simulink model "SVPWM"  (R2022a)
settings: Solver=ode23  StartTime=0.0  StopTime=0.1  MaxStep=1e-5  RelTol=1e-3
libraries: simulink x1
settings Model: Creator=123  LastModifiedBy=123

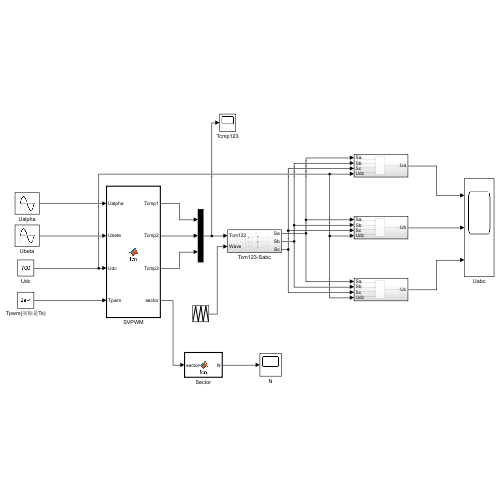
[thumbnail: Simulink's stored preview of the top-level diagram]
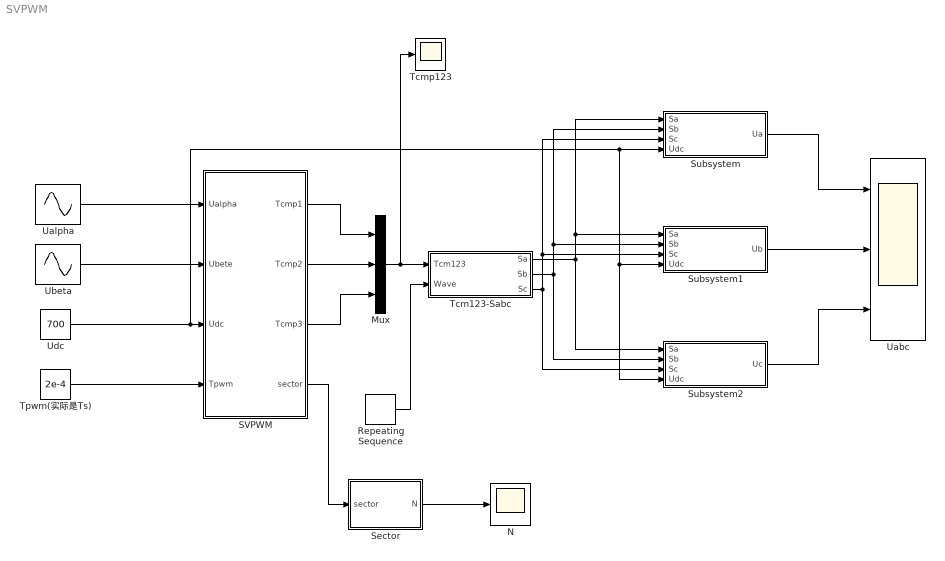
== system SVPWM ==
  Mux : Mux  Inputs=3
  N : Scope
  Repeating Sequence : simulink/Sources/Repeating Sequence  rep_seq_t=[0 0.0001 0.0002]  rep_seq_y=[0 0.0001 0]
  SVPWM : MATLAB Function  TreatAsAtomicUnit=on
  Sector : MATLAB Function  TreatAsAtomicUnit=on
  Subsystem : Subsystem
  Subsystem1 : Subsystem
  Subsystem2 : Subsystem
  Tcm123-Sabc : Subsystem
  Tcmp123 : Scope
  Tpwm(实际是Ts) : Constant  Value=2e-4
  Uabc : Scope  NumInputPorts=3
  Ualpha : Sin  Amplitude=200  Frequency=2*50*pi  Phase=pi/2  SampleTime=0
  Ubeta : Sin  Amplitude=200  Frequency=2*50*pi  SampleTime=0
  Udc : Constant  Value=700
  wires:
  Subsystem/1(Ua) -> Uabc/1
  Subsystem1/1(Ub) -> Uabc/2
  Subsystem2/1(Uc) -> Uabc/3
  Ualpha/1 -> SVPWM/1(Ualpha)
  Ubeta/1 -> SVPWM/2(Ubete)
  Udc/1 -> Subsystem/4(Udc), Subsystem1/4(Udc), Subsystem2/4(Udc), SVPWM/3(Udc)
  Tpwm(实际是Ts)/1 -> SVPWM/4(Tpwm)
  SVPWM/1(Tcmp1) -> Mux/1
  SVPWM/2(Tcmp2) -> Mux/2
  SVPWM/3(Tcmp3) -> Mux/3
  Mux/1 -> Tcmp123/1, Tcm123-Sabc/1(Tcm123)
  Repeating Sequence/1 -> Tcm123-Sabc/2(Wave)
  Tcm123-Sabc/1(Sa) -> Subsystem2/1(Sa), Subsystem1/1(Sa), Subsystem/1(Sa)
  Tcm123-Sabc/2(Sb) -> Subsystem2/2(Sb), Subsystem1/2(Sb), Subsystem/2(Sb)
  Tcm123-Sabc/3(Sc) -> Subsystem2/3(Sc), Subsystem1/3(Sc), Subsystem/3(Sc)
  SVPWM/4(sector) -> Sector/1(sector)
  Sector/1(N) -> N/1

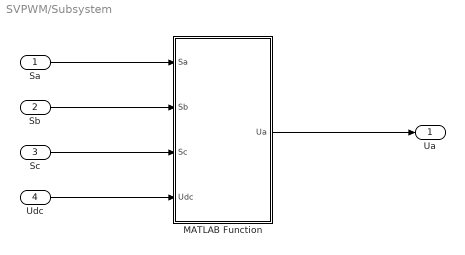
== system SVPWM/Subsystem ==
  Sa : Inport
  Sb : Inport  Port=2
  Sc : Inport  Port=3
  Udc : Inport  Port=4
  MATLAB Function : MATLAB Function  TreatAsAtomicUnit=on
  Ua : Outport
  wires:
  MATLAB Function/1(Ua) -> Ua/1
  Sa/1 -> MATLAB Function/1(Sa)
  Sb/1 -> MATLAB Function/2(Sb)
  Sc/1 -> MATLAB Function/3(Sc)
  Udc/1 -> MATLAB Function/4(Udc)

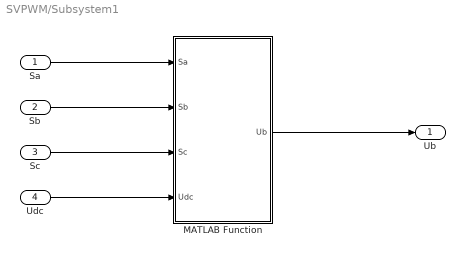
== system SVPWM/Subsystem1 ==
  Sa : Inport
  Sb : Inport  Port=2
  Sc : Inport  Port=3
  Udc : Inport  Port=4
  MATLAB Function : MATLAB Function  TreatAsAtomicUnit=on
  Ub : Outport
  wires:
  Sc/1 -> MATLAB Function/3(Sc)
  Udc/1 -> MATLAB Function/4(Udc)
  Sa/1 -> MATLAB Function/1(Sa)
  Sb/1 -> MATLAB Function/2(Sb)
  MATLAB Function/1(Ub) -> Ub/1

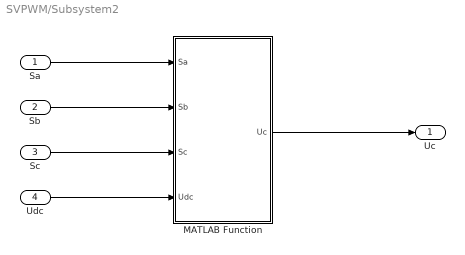
== system SVPWM/Subsystem2 ==
  Sa : Inport
  Sb : Inport  Port=2
  Sc : Inport  Port=3
  Udc : Inport  Port=4
  MATLAB Function : MATLAB Function  TreatAsAtomicUnit=on
  Uc : Outport
  wires:
  Sc/1 -> MATLAB Function/3(Sc)
  Udc/1 -> MATLAB Function/4(Udc)
  Sa/1 -> MATLAB Function/1(Sa)
  Sb/1 -> MATLAB Function/2(Sb)
  MATLAB Function/1(Uc) -> Uc/1

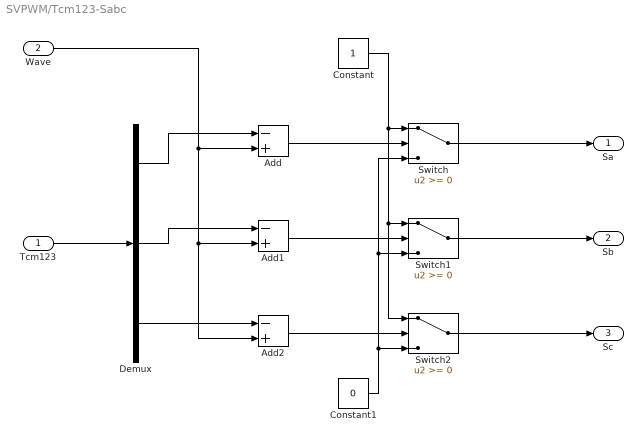
== system SVPWM/Tcm123-Sabc ==
  Tcm123 : Inport
  Wave : Inport  Port=2
  Add : Sum  Inputs=-+
  Add1 : Sum  Inputs=-+
  Add2 : Sum  Inputs=-+
  Constant : Constant
  Constant1 : Constant  Value=0
  Demux : Demux  Outputs=3
  Switch : Switch  SaturateOnIntegerOverflow=off  InputSameDT=off
  Switch1 : Switch  SaturateOnIntegerOverflow=off  InputSameDT=off
  Switch2 : Switch  SaturateOnIntegerOverflow=off  InputSameDT=off
  Sa : Outport
  Sb : Outport  Port=2
  Sc : Outport  Port=3
  wires:
  Tcm123/1 -> Demux/1
  Wave/1 -> Add/2, Add1/2, Add2/2
  Demux/1 -> Add/1
  Demux/2 -> Add1/1
  Demux/3 -> Add2/1
  Add2/1 -> Switch2/2
  Add1/1 -> Switch1/2
  Add/1 -> Switch/2
  Constant/1 -> Switch2/1, Switch1/1, Switch/1
  Constant1/1 -> Switch2/3, Switch1/3, Switch/3
  Switch/1 -> Sa/1
  Switch1/1 -> Sb/1
  Switch2/1 -> Sc/1

== matlab function SVPWM/Subsystem1/MATLAB Function ==
  data: Sa input; Ub output; Sb input; Sc input; Udc input
function Ub = fcn(Sa,Sb,Sc,Udc)

Ub = Udc/3*(2*Sb - Sa - Sc);

== matlab function SVPWM/Subsystem/MATLAB Function ==
  data: Sa input; Ua output; Sb input; Sc input; Udc input
function Ua = fcn(Sa,Sb,Sc,Udc)

Ua = Udc/3*(2*Sa - Sb - Sc);

== matlab function SVPWM/Subsystem2/MATLAB Function ==
  data: Sa input; Uc output; Sb input; Sc input; Udc input
function Uc = fcn(Sa,Sb,Sc,Udc)

Uc = Udc/3*(2*Sc - Sb - Sa);

== matlab function SVPWM/SVPWM ==
  data: Ualpha input; Tcmp1 output; Ubete input; Udc input; Tpwm input; Tcmp2 output; Tcmp3 output; sector output
function [Tcmp1,Tcmp2,Tcmp3,sector] = fcn(Ualpha,Ubete,Udc,Tpwm)

%变量初始化

Tcmp1 = 0;
Tcmp2 = 0;
Tcmp3 = 0;
sector = 0;
T1 = 0;
T2 = 0;

%扇区选择

Uref1 = Ubete;
Uref2 = (sqrt(3)*Ualpha - Ubete)/2;
Uref3 = (-sqrt(3)*Ualpha - Ubete)/2;

if(Uref1 > 0)
    sector = 1;
end
if(Uref2 > 0)
    sector = sector + 2;
end
if(Uref3 > 0)
    sector = sector + 4;
end

%非零矢量和零矢量作用时间

X = sqrt(3)*Ubete*Tpwm/Udc;
Y = Tpwm/Udc*(3/2*Ualpha + sqrt(3)/2*Ubete);
Z = Tpwm/Udc*(-3/2*Ualpha + sqrt(3)/2*Ubete);

switch(sector)
    case 1
        T1 = Z;T2 = Y;
    case 2
        T1 = Y;T2 = -X;
    case 3
        T1 = -Z;T2 = X;
    case 4
        T1 = -X;T2 = Z;
    case 5
        T1 = X;T2 = -Y;
    case 6
        T1 = -Y;T2 = -Z;
end

%过调制处理，变成占空比处理

if (T1+T2>Tpwm)
    scale = Tpwm/(T1+T2);
    T1 = T1*scale;
    T2 = T2*scale;
else
    T1 = T1;
    T2 = T2;
end

%扇区矢量切换点确定

ta = (Tpwm-(T1+T2))/4.0;
tb = ta+T1/2;
tc = tb+T2/2;

switch(sector)
    case 1
        Tcmp1 = tb;
        Tcmp2 = ta;
        Tcmp3 = tc;
    case 2
        Tcmp1 = ta;
        Tcmp2 = tc;
        Tcmp3 = tb;
    case 3
        Tcmp1 = ta;
        Tcmp2 = tb;
        Tcmp3 = tc;
    case 4
        Tcmp1 = tc;
        Tcmp2 = tb;
        Tcmp3 = ta;
    case 5
        Tcmp1 = tc;
        Tcmp2 = ta;
        Tcmp3 = tb;
    case 6
        Tcmp1 = tb;
        Tcmp2 = tc;
        Tcmp3 = ta;
end
end

== matlab function SVPWM/Sector ==
  data: sector input; N output
function N = fcn(sector)

N = 0;

switch(sector)
    case 1
        N = 2;
    case 2
        N = 6;
    case 3
        N = 1;
    case 4
        N = 4;
    case 5
        N = 3;
    case 6
        N = 5;
end
